simulink model "model_233_DirectDigital_robust"  (R2024b)
settings: Solver=FixedStepAuto  StartTime=0.0  StopTime=sIn.simulation_time  FixedStep=sIn.step_size
undefined symbols (not defined in the file): DiscIntNeverNeededParam, drv, feedback, feedback2, feedback3, gbox, mld, mot, obs, obs2, obs3, rads2rpm, rpm2rads, sens, sIn
libraries: simulink_extras x3
settings Model: Creator=bmm1  LastModifiedBy=bmm1
settings RTWCC: GPUComputeCapability=3.5

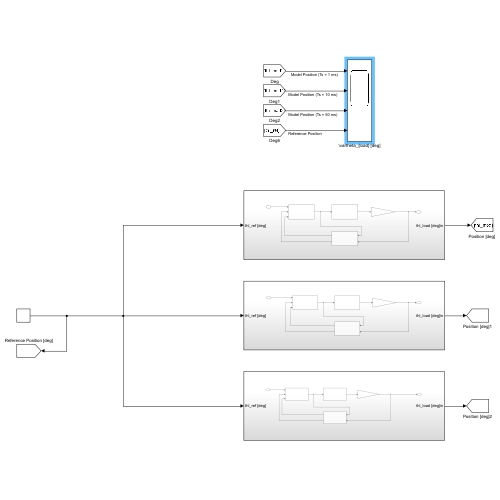
[thumbnail: Simulink's stored preview of the top-level diagram]
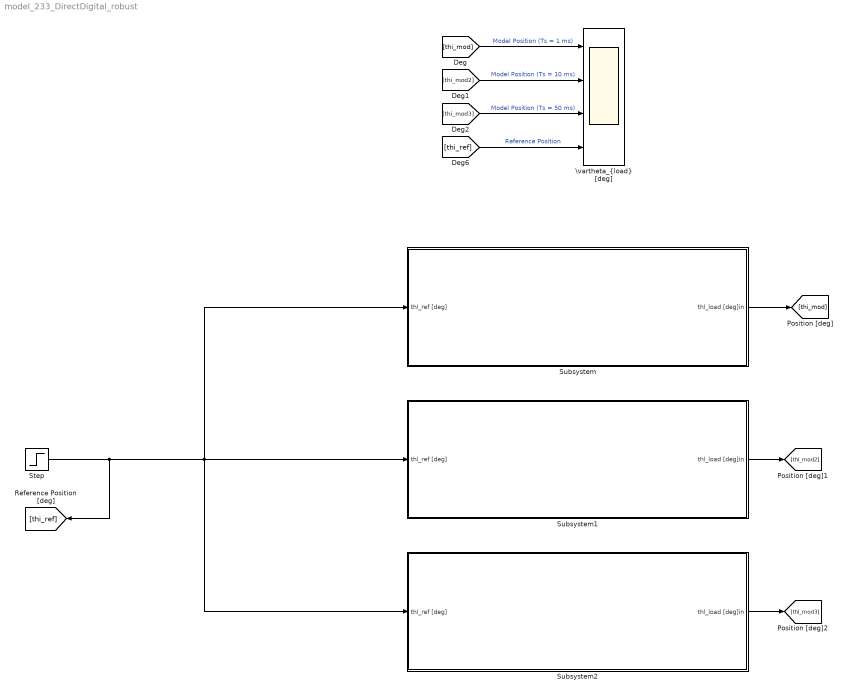
== system model_233_DirectDigital_robust ==
  Step : Step  Time=0  After=50  SampleTime=0
  Subsystem : Subsystem
  Subsystem1 : Subsystem
  Subsystem2 : Subsystem
  "\\vartheta_{load} [deg]" : Scope  NumInputPorts=4
  wires:
  [thi_mod] -> "\\vartheta_{load} [deg]"/1  "Model Position (Ts = 1 ms)"
  [thi_ref] -> "\\vartheta_{load} [deg]"/4  "Reference Position"
  Step/1 -> [thi_ref], Subsystem2/1(thl_ref [deg]), Subsystem/1(thl_ref [deg]), Subsystem1/1(thl_ref [deg])
  [thi_mod2] -> "\\vartheta_{load} [deg]"/2  "Model Position (Ts = 10 ms)"
  [thi_mod3] -> "\\vartheta_{load} [deg]"/3  "Model Position (Ts = 50 ms)"
  Subsystem/1(thl_load [deg]in) -> [thi_mod]
  Subsystem1/1(thl_load [deg]in) -> [thi_mod2]
  Subsystem2/1(thl_load [deg]in) -> [thi_mod3]

== system model_233_DirectDigital_robust/Subsystem ==
  thl_ref [deg] : Inport
  Gain : Gain  Gain=sens.enc.pulse2deg
  Selfmade model of the Quanser SRV-02 + NI DAQ : Subsystem
  State-space Controller : Subsystem
  Subsystem1 : Subsystem
  thl_load [deg]in : Outport
  wires:
  Gain/1 -> thl_load [deg]in/1, Subsystem1/2(thl_load [deg]in)
  thl_ref [deg]/1 -> State-space Controller/1(thl_ref [deg])
  State-space Controller/1(u [V]) -> Selfmade model of the Quanser SRV-02 + NI DAQ/1(u[V]), Subsystem1/1(ctr_out_u[V])
  Selfmade model of the Quanser SRV-02 + NI DAQ/1(thl[pulses]) -> Gain/1
  Subsystem1/1(thl_load [deg]Out) -> State-space Controller/3(thl [deg])
  Subsystem1/2(w_l) -> State-space Controller/2(wl [rpm])

== system model_233_DirectDigital_robust/Subsystem1 ==
  thl_ref [deg] : Inport
  Gain1 : Gain  Gain=sens.enc.pulse2deg
  Selfmade model of the Quanser SRV-02 + NI DAQ1 : Subsystem
  State-space Controller1 : Subsystem
  Subsystem3 : Subsystem
  thl_load [deg]in : Outport
  wires:
  thl_ref [deg]/1 -> State-space Controller1/1(thl_ref [deg])
  State-space Controller1/1(u [V]) -> Subsystem3/1(ctr_out_u[V]), Selfmade model of the Quanser SRV-02 + NI DAQ1/1(u[V])
  Subsystem3/1(thl_load [deg]Out) -> State-space Controller1/3(thl [deg])
  Gain1/1 -> Subsystem3/2(thl_load [deg]in), thl_load [deg]in/1
  Subsystem3/2(w_l) -> State-space Controller1/2(wl [rpm])
  Selfmade model of the Quanser SRV-02 + NI DAQ1/1(thl[pulses]) -> Gain1/1

== system model_233_DirectDigital_robust/Subsystem2 ==
  thl_ref [deg] : Inport
  Gain2 : Gain  Gain=sens.enc.pulse2deg
  Selfmade model of the Quanser SRV-02 + NI DAQ2 : Subsystem
  State-space Controller2 : Subsystem
  Subsystem3 : Subsystem
  thl_load [deg]in : Outport
  wires:
  State-space Controller2/1(u [V]) -> Selfmade model of the Quanser SRV-02 + NI DAQ2/1(u[V]), Subsystem3/1(ctr_out_u[V])
  Subsystem3/1(thl_load [deg]Out) -> State-space Controller2/3(thl [deg])
  thl_ref [deg]/1 -> State-space Controller2/1(thl_ref [deg])
  Gain2/1 -> thl_load [deg]in/1, Subsystem3/2(thl_load [deg]in)
  Subsystem3/2(w_l) -> State-space Controller2/2(wl [rpm])
  Selfmade model of the Quanser SRV-02 + NI DAQ2/1(thl[pulses]) -> Gain2/1

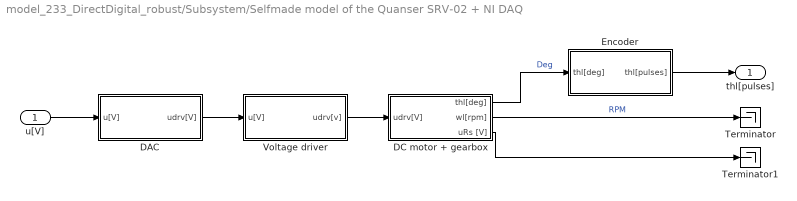
== system model_233_DirectDigital_robust/Subsystem/Selfmade model of the Quanser SRV-02 + NI DAQ ==
  u[V] : Inport
  DAC : Subsystem
  DC motor + gearbox : Subsystem
  Encoder : Subsystem
  Terminator : Terminator
  Terminator1 : Terminator
  Voltage driver : Subsystem
  thl[pulses] : Outport
  wires:
  DC motor + gearbox/1(thl[deg]) -> Encoder/1(thl[deg])  "Deg"
  u[V]/1 -> DAC/1(u[V])
  DC motor + gearbox/2(wl[rpm]) -> Terminator/1  "RPM"
  DAC/1(udrv[V]) -> Voltage driver/1(u[V])
  Voltage driver/1(udrv[v]) -> DC motor + gearbox/1(udrv[V])
  Encoder/1(thl[pulses]) -> thl[pulses]/1
  DC motor + gearbox/3(uRs [V]) -> Terminator1/1

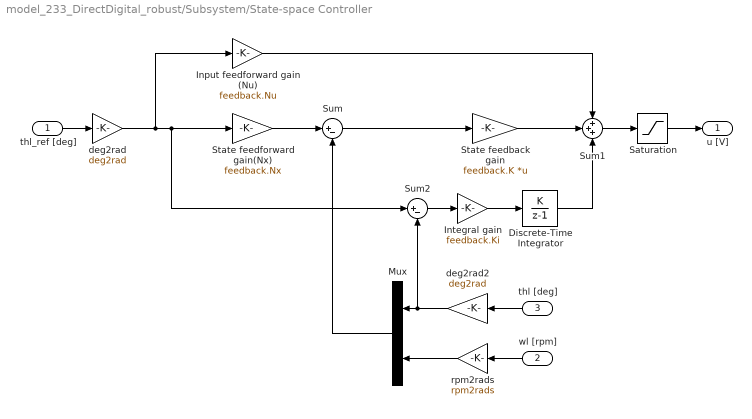
== system model_233_DirectDigital_robust/Subsystem/State-space Controller ==
  thl_ref [deg] : Inport
  wl [rpm] : Inport  Port=2
  thl [deg] : Inport  Port=3
  Discrete-Time Integrator : DiscreteIntegrator  IntegratorMethod=Accumulation: Forward Euler  SampleTime=sIn.T_s  ICPrevOutput=DiscIntNeverNeededParam  ICPrevScaledInput=DiscIntNeverNeededParam
  Input feedforward gain (Nu) : Gain  Gain=feedback.Nu
  Integral gain : Gain  Gain=feedback.Ki
  Mux : Mux  Inputs=2
  Saturation : Saturate  UpperLimit=10  LowerLimit=-10
  State feedback gain : Gain  Gain=feedback.K  Multiplication=Matrix(K*u)
  State feedforward gain(Nx) : Gain  Gain=feedback.Nx
  Sum : Sum  Inputs=|+-
  Sum1 : Sum  Inputs=+++
  Sum2 : Sum  Inputs=|+-
  deg2rad : Gain  Gain=deg2rad
  deg2rad2 : Gain  Gain=deg2rad
  rpm2rads : Gain  Gain=rpm2rads
  u [V] : Outport
  wires:
  thl_ref [deg]/1 -> deg2rad/1
  deg2rad/1 -> Input feedforward gain (Nu)/1, Sum2/1, State feedforward gain(Nx)/1
  State feedforward gain(Nx)/1 -> Sum/1
  Sum/1 -> State feedback gain/1
  State feedback gain/1 -> Sum1/2
  Input feedforward gain (Nu)/1 -> Sum1/1
  Sum1/1 -> Saturation/1
  Saturation/1 -> u [V]/1
  thl [deg]/1 -> deg2rad2/1
  wl [rpm]/1 -> rpm2rads/1
  deg2rad2/1 -> Sum2/2, Mux/1
  rpm2rads/1 -> Mux/2
  Mux/1 -> Sum/2
  Sum2/1 -> Integral gain/1
  Integral gain/1 -> Discrete-Time Integrator/1
  Discrete-Time Integrator/1 -> Sum1/3

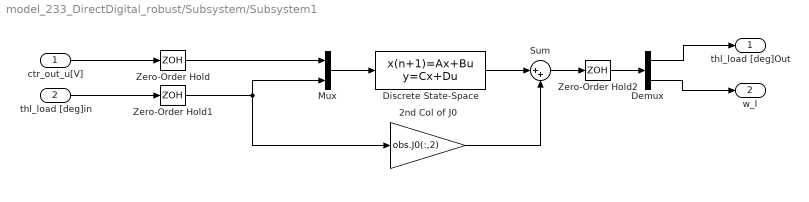
== system model_233_DirectDigital_robust/Subsystem/Subsystem1 ==
  ctr_out_u[V] : Inport
  thl_load [deg]in : Inport  Port=2
  2nd Col of J0 : Gain  Gain=obs.J0(:,2)
  Demux : Demux  Outputs=2
  Discrete State-Space : DiscreteStateSpace  A=obs.phi0  B=obs.gamma0  C=obs.H0  D=zeros(2,2)  SampleTime=sIn.T_s
  Mux : Mux  Inputs=2
  Sum : Sum  Inputs=|++
  Zero-Order Hold : ZeroOrderHold  SampleTime=sIn.T_s
  Zero-Order Hold1 : ZeroOrderHold  SampleTime=sIn.T_s
  Zero-Order Hold2 : ZeroOrderHold  SampleTime=sIn.T_s
  thl_load [deg]Out : Outport
  w_l : Outport  Port=2
  wires:
  Discrete State-Space/1 -> Sum/1
  Demux/2 -> w_l/1
  2nd Col of J0/1 -> Sum/2
  Sum/1 -> Zero-Order Hold2/1
  Demux/1 -> thl_load [deg]Out/1
  thl_load [deg]in/1 -> Zero-Order Hold1/1
  Mux/1 -> Discrete State-Space/1
  ctr_out_u[V]/1 -> Zero-Order Hold/1
  Zero-Order Hold/1 -> Mux/1
  Zero-Order Hold1/1 -> Mux/2, 2nd Col of J0/1
  Zero-Order Hold2/1 -> Demux/1

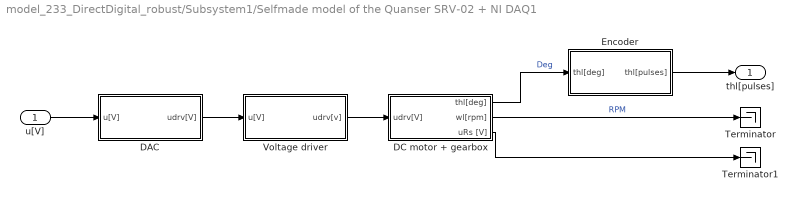
== system model_233_DirectDigital_robust/Subsystem1/Selfmade model of the Quanser SRV-02 + NI DAQ1 ==
  u[V] : Inport
  DAC : Subsystem
  DC motor + gearbox : Subsystem
  Encoder : Subsystem
  Terminator : Terminator
  Terminator1 : Terminator
  Voltage driver : Subsystem
  thl[pulses] : Outport
  wires:
  DC motor + gearbox/1(thl[deg]) -> Encoder/1(thl[deg])  "Deg"
  u[V]/1 -> DAC/1(u[V])
  DC motor + gearbox/2(wl[rpm]) -> Terminator/1  "RPM"
  DAC/1(udrv[V]) -> Voltage driver/1(u[V])
  Voltage driver/1(udrv[v]) -> DC motor + gearbox/1(udrv[V])
  Encoder/1(thl[pulses]) -> thl[pulses]/1
  DC motor + gearbox/3(uRs [V]) -> Terminator1/1

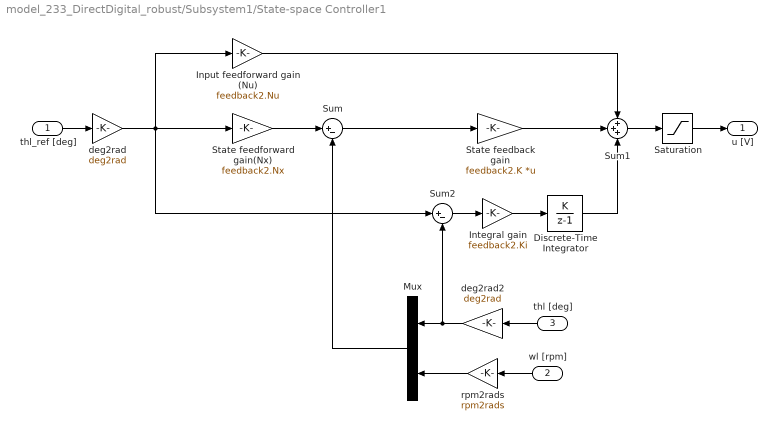
== system model_233_DirectDigital_robust/Subsystem1/State-space Controller1 ==
  thl_ref [deg] : Inport
  wl [rpm] : Inport  Port=2
  thl [deg] : Inport  Port=3
  Discrete-Time Integrator : DiscreteIntegrator  IntegratorMethod=Accumulation: Forward Euler  SampleTime=sIn.T_s2  ICPrevOutput=DiscIntNeverNeededParam  ICPrevScaledInput=DiscIntNeverNeededParam
  Input feedforward gain (Nu) : Gain  Gain=feedback2.Nu
  Integral gain : Gain  Gain=feedback2.Ki
  Mux : Mux  Inputs=2
  Saturation : Saturate  UpperLimit=10  LowerLimit=-10
  State feedback gain : Gain  Gain=feedback2.K  Multiplication=Matrix(K*u)
  State feedforward gain(Nx) : Gain  Gain=feedback2.Nx
  Sum : Sum  Inputs=|+-
  Sum1 : Sum  Inputs=+++
  Sum2 : Sum  Inputs=|+-
  deg2rad : Gain  Gain=deg2rad
  deg2rad2 : Gain  Gain=deg2rad
  rpm2rads : Gain  Gain=rpm2rads
  u [V] : Outport
  wires:
  thl_ref [deg]/1 -> deg2rad/1
  State feedforward gain(Nx)/1 -> Sum/1
  Sum/1 -> State feedback gain/1
  State feedback gain/1 -> Sum1/2
  Input feedforward gain (Nu)/1 -> Sum1/1
  Sum1/1 -> Saturation/1
  Saturation/1 -> u [V]/1
  thl [deg]/1 -> deg2rad2/1
  wl [rpm]/1 -> rpm2rads/1
  rpm2rads/1 -> Mux/2
  Mux/1 -> Sum/2
  deg2rad/1 -> Sum2/1, Input feedforward gain (Nu)/1, State feedforward gain(Nx)/1
  Integral gain/1 -> Discrete-Time Integrator/1
  Discrete-Time Integrator/1 -> Sum1/3
  Sum2/1 -> Integral gain/1
  deg2rad2/1 -> Sum2/2, Mux/1

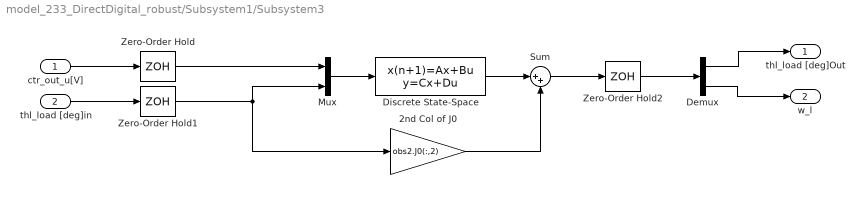
== system model_233_DirectDigital_robust/Subsystem1/Subsystem3 ==
  ctr_out_u[V] : Inport
  thl_load [deg]in : Inport  Port=2
  2nd Col of J0 : Gain  Gain=obs2.J0(:,2)
  Demux : Demux  Outputs=2
  Discrete State-Space : DiscreteStateSpace  A=obs2.phi0  B=obs2.gamma0  C=obs2.H0  D=zeros(2,2)  SampleTime=sIn.T_s2
  Mux : Mux  Inputs=2
  Sum : Sum  Inputs=|++
  Zero-Order Hold : ZeroOrderHold  SampleTime=sIn.T_s2
  Zero-Order Hold1 : ZeroOrderHold  SampleTime=sIn.T_s2
  Zero-Order Hold2 : ZeroOrderHold  SampleTime=sIn.T_s2
  thl_load [deg]Out : Outport
  w_l : Outport  Port=2
  wires:
  Discrete State-Space/1 -> Sum/1
  Demux/2 -> w_l/1
  2nd Col of J0/1 -> Sum/2
  Sum/1 -> Zero-Order Hold2/1
  Demux/1 -> thl_load [deg]Out/1
  thl_load [deg]in/1 -> Zero-Order Hold1/1
  Mux/1 -> Discrete State-Space/1
  ctr_out_u[V]/1 -> Zero-Order Hold/1
  Zero-Order Hold/1 -> Mux/1
  Zero-Order Hold1/1 -> Mux/2, 2nd Col of J0/1
  Zero-Order Hold2/1 -> Demux/1

== system model_233_DirectDigital_robust/Subsystem2/Selfmade model of the Quanser SRV-02 + NI DAQ2 ==
  u[V] : Inport
  DAC : Subsystem
  DC motor + gearbox : Subsystem
  Encoder : Subsystem
  Terminator : Terminator
  Terminator1 : Terminator
  Voltage driver : Subsystem
  thl[pulses] : Outport
  wires:
  DC motor + gearbox/1(thl[deg]) -> Encoder/1(thl[deg])  "Deg"
  u[V]/1 -> DAC/1(u[V])
  DC motor + gearbox/2(wl[rpm]) -> Terminator/1  "RPM"
  DAC/1(udrv[V]) -> Voltage driver/1(u[V])
  Voltage driver/1(udrv[v]) -> DC motor + gearbox/1(udrv[V])
  Encoder/1(thl[pulses]) -> thl[pulses]/1
  DC motor + gearbox/3(uRs [V]) -> Terminator1/1

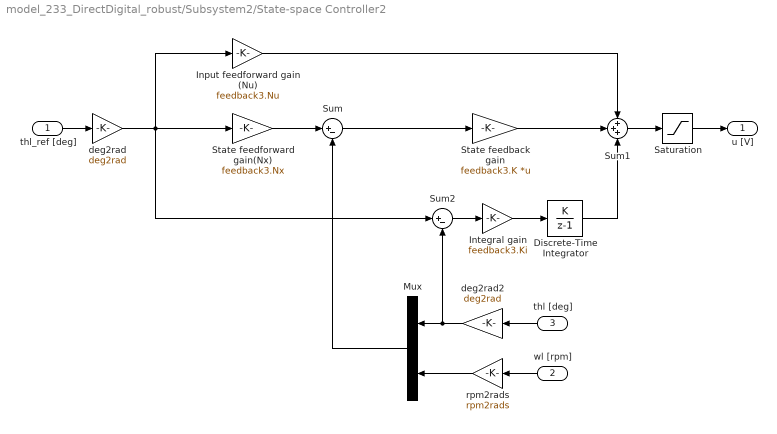
== system model_233_DirectDigital_robust/Subsystem2/State-space Controller2 ==
  thl_ref [deg] : Inport
  wl [rpm] : Inport  Port=2
  thl [deg] : Inport  Port=3
  Discrete-Time Integrator : DiscreteIntegrator  IntegratorMethod=Accumulation: Forward Euler  SampleTime=sIn.T_s3  ICPrevOutput=DiscIntNeverNeededParam  ICPrevScaledInput=DiscIntNeverNeededParam
  Input feedforward gain (Nu) : Gain  Gain=feedback3.Nu
  Integral gain : Gain  Gain=feedback3.Ki
  Mux : Mux  Inputs=2
  Saturation : Saturate  UpperLimit=10  LowerLimit=-10
  State feedback gain : Gain  Gain=feedback3.K  Multiplication=Matrix(K*u)
  State feedforward gain(Nx) : Gain  Gain=feedback3.Nx
  Sum : Sum  Inputs=|+-
  Sum1 : Sum  Inputs=+++
  Sum2 : Sum  Inputs=|+-
  deg2rad : Gain  Gain=deg2rad
  deg2rad2 : Gain  Gain=deg2rad
  rpm2rads : Gain  Gain=rpm2rads
  u [V] : Outport
  wires:
  thl_ref [deg]/1 -> deg2rad/1
  State feedforward gain(Nx)/1 -> Sum/1
  Sum/1 -> State feedback gain/1
  State feedback gain/1 -> Sum1/2
  Input feedforward gain (Nu)/1 -> Sum1/1
  Sum1/1 -> Saturation/1
  Saturation/1 -> u [V]/1
  thl [deg]/1 -> deg2rad2/1
  wl [rpm]/1 -> rpm2rads/1
  rpm2rads/1 -> Mux/2
  Mux/1 -> Sum/2
  deg2rad/1 -> Sum2/1, Input feedforward gain (Nu)/1, State feedforward gain(Nx)/1
  Integral gain/1 -> Discrete-Time Integrator/1
  Discrete-Time Integrator/1 -> Sum1/3
  Sum2/1 -> Integral gain/1
  deg2rad2/1 -> Sum2/2, Mux/1

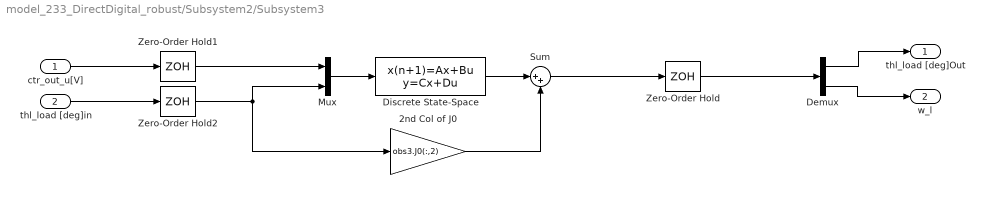
== system model_233_DirectDigital_robust/Subsystem2/Subsystem3 ==
  ctr_out_u[V] : Inport
  thl_load [deg]in : Inport  Port=2
  2nd Col of J0 : Gain  Gain=obs3.J0(:,2)
  Demux : Demux  Outputs=2
  Discrete State-Space : DiscreteStateSpace  A=obs3.phi0  B=obs3.gamma0  C=obs3.H0  D=zeros(2,2)  SampleTime=sIn.T_s3
  Mux : Mux  Inputs=2
  Sum : Sum  Inputs=|++
  Zero-Order Hold : ZeroOrderHold  SampleTime=sIn.T_s3
  Zero-Order Hold1 : ZeroOrderHold  SampleTime=sIn.T_s3
  Zero-Order Hold2 : ZeroOrderHold  SampleTime=sIn.T_s3
  thl_load [deg]Out : Outport
  w_l : Outport  Port=2
  wires:
  Discrete State-Space/1 -> Sum/1
  Demux/2 -> w_l/1
  2nd Col of J0/1 -> Sum/2
  Demux/1 -> thl_load [deg]Out/1
  thl_load [deg]in/1 -> Zero-Order Hold2/1
  Mux/1 -> Discrete State-Space/1
  ctr_out_u[V]/1 -> Zero-Order Hold1/1
  Sum/1 -> Zero-Order Hold/1
  Zero-Order Hold1/1 -> Mux/1
  Zero-Order Hold2/1 -> Mux/2, 2nd Col of J0/1
  Zero-Order Hold/1 -> Demux/1

== system model_233_DirectDigital_robust/Subsystem/Selfmade model of the Quanser SRV-02 + NI DAQ/DAC ==
  u[V] : Inport
  Quantizer : Quantizer  QuantizationInterval=daq.dac.q
  Saturation : Saturate  UpperLimit=10  LowerLimit=-10
  Zero-Order Hold : ZeroOrderHold  SampleTime=1e-3
  udrv[V] : Outport
  wires:
  Zero-Order Hold/1 -> Quantizer/1
  u[V]/1 -> Zero-Order Hold/1
  Quantizer/1 -> Saturation/1
  Saturation/1 -> udrv[V]/1

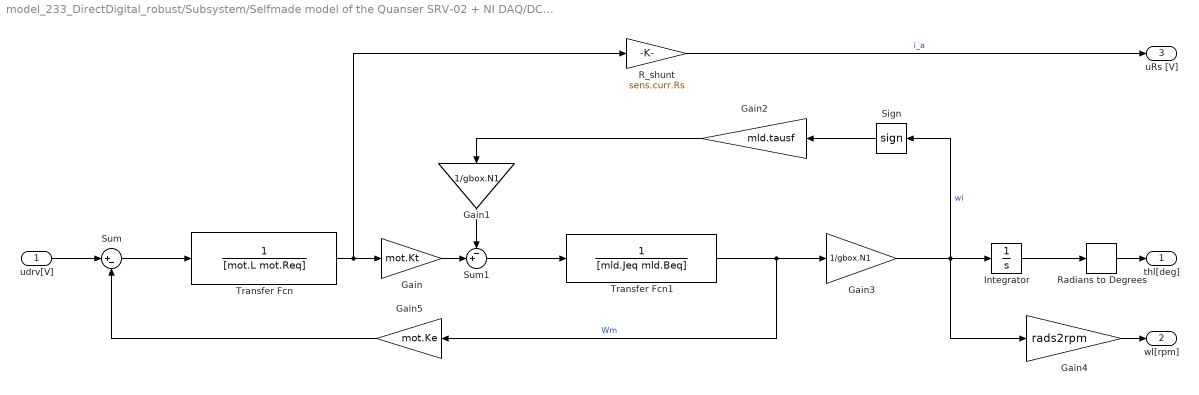
== system model_233_DirectDigital_robust/Subsystem/Selfmade model of the Quanser SRV-02 + NI DAQ/DC motor + gearbox ==
  udrv[V] : Inport
  Gain : Gain  Gain=mot.Kt
  Gain1 : Gain  Gain=1/gbox.N1
  Gain2 : Gain  Gain=mld.tausf
  Gain3 : Gain  Gain=1/gbox.N1
  Gain4 : Gain  Gain=rads2rpm
  Gain5 : Gain  Gain=mot.Ke
  Integrator : Integrator
  R_shunt : Gain  Gain=sens.curr.Rs
  Radians to Degrees : simulink_extras/Transformations/Radians to Degrees
  Sign : Signum  ZeroCross=off
  Sum : Sum  Inputs=|+-
  Sum1 : Sum  Inputs=-+|
  Transfer Fcn : TransferFcn  Denominator=[mot.L mot.Req]
  Transfer Fcn1 : TransferFcn  Denominator=[mld.Jeq mld.Beq]
  thl[deg] : Outport
  wl[rpm] : Outport  Port=2
  uRs [V] : Outport  Port=3
  wires:
  udrv[V]/1 -> Sum/1
  Sum/1 -> Transfer Fcn/1
  Transfer Fcn/1 -> R_shunt/1, Gain/1
  Gain1/1 -> Sum1/1
  Gain2/1 -> Gain1/1
  Sign/1 -> Gain2/1
  Transfer Fcn1/1 -> Gain5/1, Gain3/1  "Wm"
  Gain3/1 -> Gain4/1, Sign/1, Integrator/1  "wl"
  Integrator/1 -> Radians to Degrees/1
  Radians to Degrees/1 -> thl[deg]/1
  Gain4/1 -> wl[rpm]/1
  Sum1/1 -> Transfer Fcn1/1
  Gain/1 -> Sum1/2
  Gain5/1 -> Sum/2
  R_shunt/1 -> uRs [V]/1  "i_a"

== system model_233_DirectDigital_robust/Subsystem/Selfmade model of the Quanser SRV-02 + NI DAQ/Encoder ==
  thl[deg] : Inport
  Gain : Gain  Gain=1/sens.enc.pulse2deg
  Quantizer : Quantizer  QuantizationInterval=sens.enc.pulse2deg
  Zero-Order Hold : ZeroOrderHold  SampleTime=1e-3
  thl[pulses] : Outport
  wires:
  thl[deg]/1 -> Zero-Order Hold/1
  Gain/1 -> thl[pulses]/1
  Quantizer/1 -> Gain/1
  Zero-Order Hold/1 -> Quantizer/1

== system model_233_DirectDigital_robust/Subsystem/Selfmade model of the Quanser SRV-02 + NI DAQ/Voltage driver ==
  u[V] : Inport
  Saturation : Saturate  UpperLimit=12  LowerLimit=-12
  Transfer Fcn : TransferFcn  Numerator=[drv.dcgain]  Denominator=[drv.Tc 1]
  udrv[v] : Outport
  wires:
  u[V]/1 -> Transfer Fcn/1
  Transfer Fcn/1 -> Saturation/1
  Saturation/1 -> udrv[v]/1

== system model_233_DirectDigital_robust/Subsystem1/Selfmade model of the Quanser SRV-02 + NI DAQ1/DAC ==
  u[V] : Inport
  Quantizer : Quantizer  QuantizationInterval=daq.dac.q
  Saturation : Saturate  UpperLimit=10  LowerLimit=-10
  Zero-Order Hold : ZeroOrderHold  SampleTime=1e-3
  udrv[V] : Outport
  wires:
  Zero-Order Hold/1 -> Quantizer/1
  u[V]/1 -> Zero-Order Hold/1
  Quantizer/1 -> Saturation/1
  Saturation/1 -> udrv[V]/1

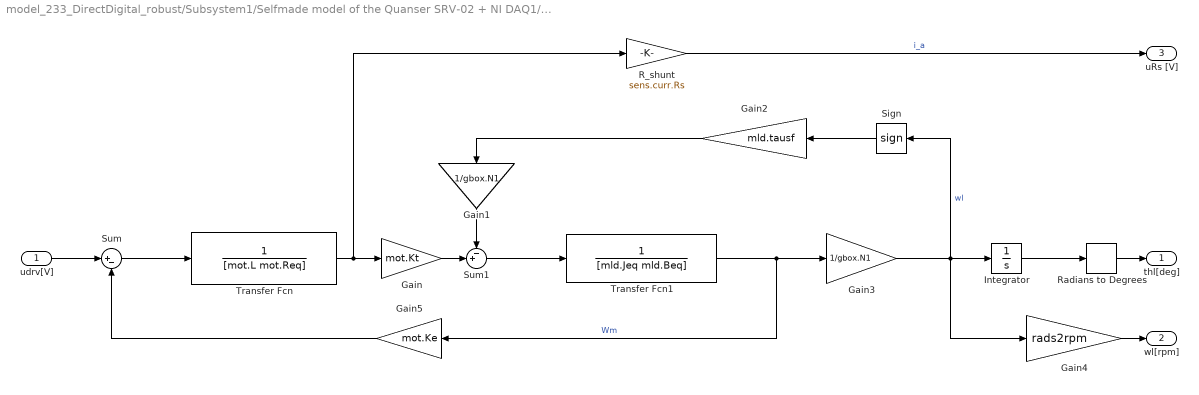
== system model_233_DirectDigital_robust/Subsystem1/Selfmade model of the Quanser SRV-02 + NI DAQ1/DC motor + gearbox ==
  udrv[V] : Inport
  Gain : Gain  Gain=mot.Kt
  Gain1 : Gain  Gain=1/gbox.N1
  Gain2 : Gain  Gain=mld.tausf
  Gain3 : Gain  Gain=1/gbox.N1
  Gain4 : Gain  Gain=rads2rpm
  Gain5 : Gain  Gain=mot.Ke
  Integrator : Integrator
  R_shunt : Gain  Gain=sens.curr.Rs
  Radians to Degrees : simulink_extras/Transformations/Radians to Degrees
  Sign : Signum  ZeroCross=off
  Sum : Sum  Inputs=|+-
  Sum1 : Sum  Inputs=-+|
  Transfer Fcn : TransferFcn  Denominator=[mot.L mot.Req]
  Transfer Fcn1 : TransferFcn  Denominator=[mld.Jeq mld.Beq]
  thl[deg] : Outport
  wl[rpm] : Outport  Port=2
  uRs [V] : Outport  Port=3
  wires:
  udrv[V]/1 -> Sum/1
  Sum/1 -> Transfer Fcn/1
  Transfer Fcn/1 -> R_shunt/1, Gain/1
  Gain1/1 -> Sum1/1
  Gain2/1 -> Gain1/1
  Sign/1 -> Gain2/1
  Transfer Fcn1/1 -> Gain5/1, Gain3/1  "Wm"
  Gain3/1 -> Gain4/1, Sign/1, Integrator/1  "wl"
  Integrator/1 -> Radians to Degrees/1
  Radians to Degrees/1 -> thl[deg]/1
  Gain4/1 -> wl[rpm]/1
  Sum1/1 -> Transfer Fcn1/1
  Gain/1 -> Sum1/2
  Gain5/1 -> Sum/2
  R_shunt/1 -> uRs [V]/1  "i_a"

== system model_233_DirectDigital_robust/Subsystem1/Selfmade model of the Quanser SRV-02 + NI DAQ1/Encoder ==
  thl[deg] : Inport
  Gain : Gain  Gain=1/sens.enc.pulse2deg
  Quantizer : Quantizer  QuantizationInterval=sens.enc.pulse2deg
  Zero-Order Hold : ZeroOrderHold  SampleTime=1e-3
  thl[pulses] : Outport
  wires:
  thl[deg]/1 -> Zero-Order Hold/1
  Gain/1 -> thl[pulses]/1
  Quantizer/1 -> Gain/1
  Zero-Order Hold/1 -> Quantizer/1

== system model_233_DirectDigital_robust/Subsystem1/Selfmade model of the Quanser SRV-02 + NI DAQ1/Voltage driver ==
  u[V] : Inport
  Saturation : Saturate  UpperLimit=12  LowerLimit=-12
  Transfer Fcn : TransferFcn  Numerator=[drv.dcgain]  Denominator=[drv.Tc 1]
  udrv[v] : Outport
  wires:
  u[V]/1 -> Transfer Fcn/1
  Transfer Fcn/1 -> Saturation/1
  Saturation/1 -> udrv[v]/1

== system model_233_DirectDigital_robust/Subsystem2/Selfmade model of the Quanser SRV-02 + NI DAQ2/DAC ==
  u[V] : Inport
  Quantizer : Quantizer  QuantizationInterval=daq.dac.q
  Saturation : Saturate  UpperLimit=10  LowerLimit=-10
  Zero-Order Hold : ZeroOrderHold  SampleTime=1e-3
  udrv[V] : Outport
  wires:
  Zero-Order Hold/1 -> Quantizer/1
  u[V]/1 -> Zero-Order Hold/1
  Quantizer/1 -> Saturation/1
  Saturation/1 -> udrv[V]/1

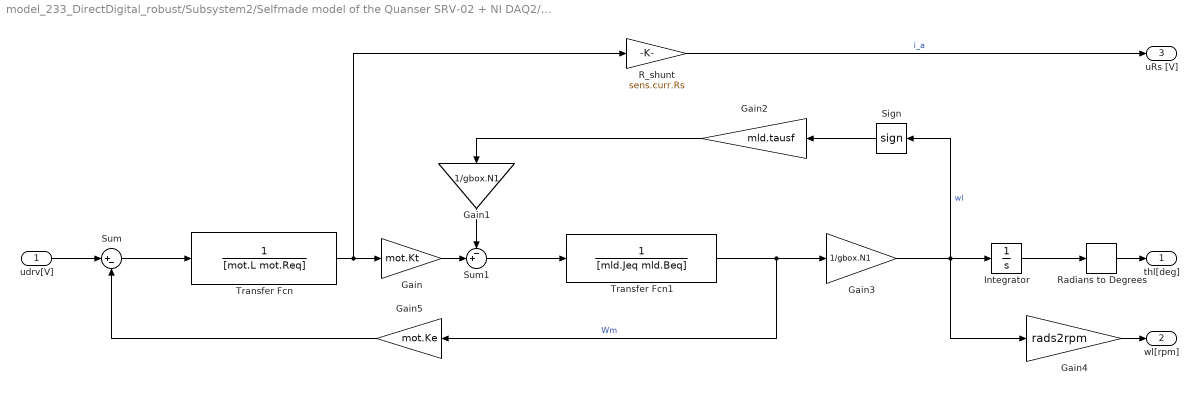
== system model_233_DirectDigital_robust/Subsystem2/Selfmade model of the Quanser SRV-02 + NI DAQ2/DC motor + gearbox ==
  udrv[V] : Inport
  Gain : Gain  Gain=mot.Kt
  Gain1 : Gain  Gain=1/gbox.N1
  Gain2 : Gain  Gain=mld.tausf
  Gain3 : Gain  Gain=1/gbox.N1
  Gain4 : Gain  Gain=rads2rpm
  Gain5 : Gain  Gain=mot.Ke
  Integrator : Integrator
  R_shunt : Gain  Gain=sens.curr.Rs
  Radians to Degrees : simulink_extras/Transformations/Radians to Degrees
  Sign : Signum  ZeroCross=off
  Sum : Sum  Inputs=|+-
  Sum1 : Sum  Inputs=-+|
  Transfer Fcn : TransferFcn  Denominator=[mot.L mot.Req]
  Transfer Fcn1 : TransferFcn  Denominator=[mld.Jeq mld.Beq]
  thl[deg] : Outport
  wl[rpm] : Outport  Port=2
  uRs [V] : Outport  Port=3
  wires:
  udrv[V]/1 -> Sum/1
  Sum/1 -> Transfer Fcn/1
  Transfer Fcn/1 -> R_shunt/1, Gain/1
  Gain1/1 -> Sum1/1
  Gain2/1 -> Gain1/1
  Sign/1 -> Gain2/1
  Transfer Fcn1/1 -> Gain5/1, Gain3/1  "Wm"
  Gain3/1 -> Gain4/1, Sign/1, Integrator/1  "wl"
  Integrator/1 -> Radians to Degrees/1
  Radians to Degrees/1 -> thl[deg]/1
  Gain4/1 -> wl[rpm]/1
  Sum1/1 -> Transfer Fcn1/1
  Gain/1 -> Sum1/2
  Gain5/1 -> Sum/2
  R_shunt/1 -> uRs [V]/1  "i_a"

== system model_233_DirectDigital_robust/Subsystem2/Selfmade model of the Quanser SRV-02 + NI DAQ2/Encoder ==
  thl[deg] : Inport
  Gain : Gain  Gain=1/sens.enc.pulse2deg
  Quantizer : Quantizer  QuantizationInterval=sens.enc.pulse2deg
  Zero-Order Hold : ZeroOrderHold  SampleTime=1e-3
  thl[pulses] : Outport
  wires:
  thl[deg]/1 -> Zero-Order Hold/1
  Gain/1 -> thl[pulses]/1
  Quantizer/1 -> Gain/1
  Zero-Order Hold/1 -> Quantizer/1

== system model_233_DirectDigital_robust/Subsystem2/Selfmade model of the Quanser SRV-02 + NI DAQ2/Voltage driver ==
  u[V] : Inport
  Saturation : Saturate  UpperLimit=12  LowerLimit=-12
  Transfer Fcn : TransferFcn  Numerator=[drv.dcgain]  Denominator=[drv.Tc 1]
  udrv[v] : Outport
  wires:
  u[V]/1 -> Transfer Fcn/1
  Transfer Fcn/1 -> Saturation/1
  Saturation/1 -> udrv[v]/1
